simulink model "untitled"  (R2022a)
settings: Solver=VariableStepAuto  StartTime=0.0  StopTime=10  RelTol=1e-3
values from neighbouring files (symbols this model uses):
  C_PM = 1.758e-3    (= 0.001758)    [journal.m]
  Cfilter = 1/(Larm*wc2)    (= 4.78421193241e-05)    [journal.m]
  Cg = 50e-9    (= 5e-08)    [journal.m]
  Fc = Fnom*3.37    (= 168.5)    [journal.m]
  Fnom = 50    [journal.m]
  Inom = Pnom/(sqrt(3)*Vnom_dc)    [journal.m]
  Ki_Ireg = 6    [journal.m]
  Ki_Preg = 1.0    (= 1)    [journal.m]
  Ki_Qreg = 1.0    (= 1)    [journal.m]
  Ki_VDCreg = 100    [journal.m]
  Kp_Ireg = 0.6    [journal.m]
  Kp_Preg = 0.5/3    (= 0.166666666667)    [journal.m]
  Kp_Qreg = 0.5/3    (= 0.166666666667)    [journal.m]
  Kp_VDCreg = 4    [journal.m]
  L_cable = 15e-3    (= 0.015)    [journal.m]
  Larm = Larm_pu*(Zbase/(2*pi*Fnom))    (= 0.0529455974536)    [journal.m]
  Lff = Larm_pu/2    (= 0.075)    [journal.m]
  Lfilter = 0    [journal.m]
  Limits_Ireg = [ 2.0  -2.0]    [journal.m]
  Limits_Preg = [ 1.2, 0.8 ]    [journal.m]
  Limits_Qreg = [ 0.25, -0.25 ]    [journal.m]
  Limits_VDCreg = [ 2.0  -2.0]    [journal.m]
  Lxfo = 0.12    [journal.m]
  Nb_PM = 36    [journal.m]
  Pnom = 1000e6    (= 1000000000)    [journal.m]
  R_cable = 0.5    [journal.m]
  R_startup = 400    [journal.m]
  Rarm = Rarm_pu*Zbase    (= 0.1663335)    [journal.m]
  Rff = Rarm_pu/2    (= 0.00075)    [journal.m]
  Rfilter = 1/(Cfilter*w)*30    (= 1996.002)    [journal.m]
  Rg = 100    [journal.m]
  Rxfo = 0.003    [journal.m]
  Slope_Pref = 0.5    [journal.m]
  Slope_Qref = 0.5    [journal.m]
  Slope_Vdc_ref = Vnom_dc/5    (= 128000)    [journal.m]
  Tbrk1_On = 0.1    [journal.m]
  Tbrk2_On = 0.5    [journal.m]
  Tdeblock = 1    [journal.m]
  Tfault = 999    [journal.m]
  Ton_Converter2 = 2    [journal.m]
  Ton_PQreg = 2    [journal.m]
  Ton_VDCreg = 1    [journal.m]
  Ts = Ts_Control    (= 4e-05)    [journal.m]
  Ts_Control = 40e-6    (= 4e-05)    [journal.m]
  Ts_Power = 20e-6    (= 2e-05)    [journal.m]
  Vnom_dc = 640e3    (= 640000)    [journal.m]
  Vnom_prim = 400e3    (= 400000)    [journal.m]
  Vnom_sec = 333e3    (= 333000)    [journal.m]
undefined symbols (not defined in the file or in its folder): D11, Delta, DiscIntNeverNeededParam, find_system, Pcc, sigbuilder_block
libraries: powerlib_extras x42, spsSeriesRLCBranchLib x32, spsCurrentMeasurementLib x24, simulink x18, spsVoltageMeasurementLib x16, spsHalfBridgeMMCLib x12, spsThreePhaseVIMeasurementLib x10, simulink_extras x6, spsBreakerLib x6, spsParallelRLCBranchLib x6, spsThreePhaseBreakerLib x4, spsMeanLib x4
(part 1 of 6)
settings Model: SimulationMode=accelerator  Creator=Hai  LastModifiedBy=Hai

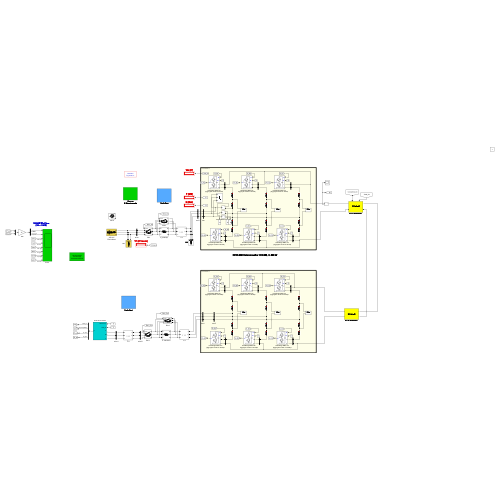
[thumbnail: Simulink's stored preview of the top-level diagram]
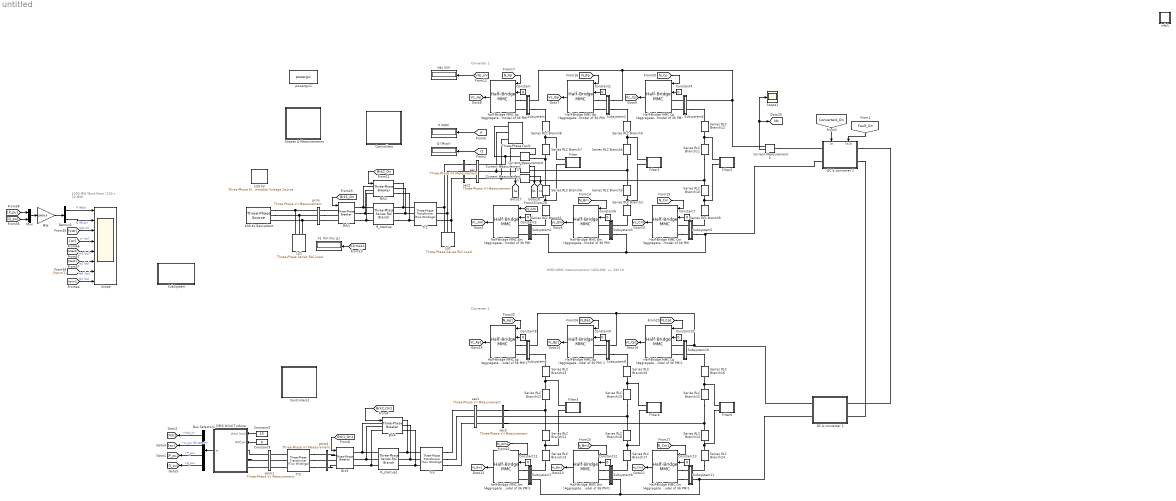
== system untitled ==
  note: HVDC-MMC Interconnection 1000-MW, +/- 320 kV
  note: Converter 1
  note: Converter 1
  note: 1000 MW Wind Farm
      | (100 x 10 MW)
  120 kV : spsThreePhaseProgrammableVoltageSourceLib/Three-Phase Programmable Voltage Source  PositiveSequence=[400e3 0 50]  VariationEntity=Amplitude  VariationType=Table of time-amplitude pairs  VariationTypeAlt=Step  VariationStep=-0.2  VariationRate=10  VariationMagnitude=0.3  VariationFrequency=2  VariationTiming=[0.05 0.05+5/60]  VariationPhaseA=off  Amplitudes=[1 0.4 1.0]  TimeValues=[0 7 7.5]  HarmonicGeneration=off  HarmonicA=[1 -0.1 0 2]  HarmonicB=[2 0.15 35 2]*0  Timing="[0.1  2]"  BusType=swing  Pref=0  Qref=0  Qmin=-inf  Qmax=inf
  400-kV Equivalent : spsThreePhaseSourceLib/Three-Phase Source  InternalConnection=Yg  VoltagePhases=off  Voltage=Vnom_prim*0.99  PhaseAngle=0  Voltage_phases=[25e3 25e3 25e3]/sqrt(3)  PhaseAngles_phases=[0 -120 +120]  Frequency=Fnom  NonIdealSource=on  SpecifyImpedance=on  Resistance=0.8929  Inductance=16.58e-3  ShortCircuitLevel=Psc  BaseVoltage=Vnom_prim  XRratio=7  BusType=swing  Pref=0  Qref=0  Prefabc=[10e3, 10e3, 10e3]  Qrefabc=[0, 0, 0]  Qmin=-inf  Qmax=inf
  Brk1 : spsThreePhaseBreakerLib/Three-Phase Breaker  InitialState=open  SwitchA=on  SwitchB=on  SwitchC=on  SwitchTimes=0.1  External=on  BreakerResistance=0.001  SnubberResistance=1e6  SnubberCapacitance=inf  Measurements=None
  Brk2 : spsThreePhaseBreakerLib/Three-Phase Breaker  InitialState=open  SwitchA=on  SwitchB=on  SwitchC=on  SwitchTimes=[30/60]*10000  External=on  BreakerResistance=0.01  SnubberResistance=1e6  SnubberCapacitance=inf  Measurements=None
  Brk3 : spsThreePhaseBreakerLib/Three-Phase Breaker  InitialState=open  SwitchA=on  SwitchB=on  SwitchC=on  SwitchTimes=0.1  External=on  BreakerResistance=0.001  SnubberResistance=1e6  SnubberCapacitance=inf  Measurements=None
  Brk4 : spsThreePhaseBreakerLib/Three-Phase Breaker  InitialState=open  SwitchA=on  SwitchB=on  SwitchC=on  SwitchTimes=[30/60]*10000  External=on  BreakerResistance=0.01  SnubberResistance=1e6  SnubberCapacitance=inf  Measurements=None
  Bus Selector1 : BusSelector  OutputSignals=Vdc_V,wr_pu (IG speed),PQ_pu.P_pu,PQ_pu.Q_pu
  Constant{,1,3..13} (13 alike) : Constant  Value=0
  Constant2 : Constant  Value=15
  Controllers : Subsystem
  Controllers1 : Subsystem
  Current Measurement{,1..3} (4 alike) : spsCurrentMeasurementLib/Current Measurement  PhasorSimulation=off  OutputType=Complex  PSBequivalent=0
  DC & converter 1 : Subsystem
      mask Display: disp('DC circuit')
  DC & converter 2 : Subsystem
      settings: PortSchema="{\"entries\":[{\"content\":{\"sides\":[{\"content\":{\"connectorIds\":[\"LConn1\",\"LConn2\"]},\"type\":\"ConnectorPlacement.EquallySpacedRectSide\",\"uuid\":\"7a2c87ad-91de-4512-ad2a-35713ffc2c67\"},{\"content\":{\"connectorIds\":[\"RConn1\",\"RConn2\"],\"side\":\"RIGHT\"},\"type\":\"ConnectorPlacement.EquallySpacedRectSide\",\"uuid\":\"a4d51b8d-9b80-4f56-8990-d227af10d4d9\"},{\"content\":{\"connectorIds\":[\"In1\",\"In2\"],\"side\":\"TOP\"},\"type\":\"ConnectorPlacement.EquallySpacedRectSide\",\"uuid\":\"21e823e1-439d-404c-83ef-6279f9df48a0\"}]},\"type\":\"ConnectorPlacement.EquallySpacedConnector\",\"uuid\":\"7be36849-7bc6-4892-aa95-a5e675f45e41\"}],\"packageUris\":[\"http://schema.mathworks.com/mf0/Connector/R2020b\"],\"version\":\"1.0\"}"
      mask Display: disp('DC circuit')
  DFIG Wind Turbine : Subsystem  LoadFcn=%find_system(gcs,'FollowLinks', 'on', 'LookUnderMasks', 'all');  mask(DFIG Wind Turbine){Nb_wt=666, ShowParameters=Generator data for 1 wind turbine, nom=[1.5e6/.9 575 1975 50], sta=[ 0.023 0.18], rot=[ 0.016 0.16], Lm=2.9, mec=[0.685 0.01 3], init=[ -0.2,0   0,0,0   0,0,0 ], Imax_grid_conv=0.8, RL_grid=[ 0.3 0.003], Vdc_nom=1150, C_DClink1=10000e-6, C_var_filter1=120e3, Pmec1=1.5e6, wind_speed_CpMax=11, wind0=11, DisplayTurbChar=off, H_WT=4.32, Ksh=1.11, D_mutual=1.5, w_wt0=1.2, torque0=0.83, Kdc=[8   400], Kgrid_side_cur_reg=[0.83 5], Kspeed=[3 0.6], Krotor_side_cur_reg=[0.6 8], Ki_QV=[0.05 20], Kp_pitch=[150], Kcompensation=[3 30], pitch_max=27, pitch_rate=10}
      mask prompts: Nb_wt "Number of wind turbines:"; ShowParameters "Display:"; nom "Nom. power, L-L volt. and freq. [Pn (VA), Vs_nom (Vrms), Vr_nom (Vrms), fn (Hz)]:"; sta "Stator [ Rs,Lls ] (p.u.):"; rot "Rotor [ Rr',Llr' ] (p.u.):"; Lm "Magnetizing inductance Lm (p.u.):"; mec "Inertia constant, friction factor, and pairs of poles [ H(s)  F(p.u.)  p ]:"; init "Initial conditions [s  th  ias  ibs  ics  phaseas phasebs phasecs]:"; Imax_grid_conv "Grid-side converter maximum current (pu of generator nominal current):"; RL_grid "Grid-side coupling inductor [ L, R] (p.u.):"; Vdc_nom "Nominal DC bus voltage (V):"; C_DClink1 "DC bus capacitor (F):"; C_var_filter1 "Line filter capacitor (Q=50) (var):"; Pmec1 "Nominal mechanical output power (W):"; wind_speed_CpMax "Wind speed at nominal speed and at Cp max (must be between 6 m/s and 30 m/s) (m/s):"; wind0 "Initial wind speed (m/s):"; DisplayTurbChar "Display wind turbine power characteristics:"; H_WT "Wind turbine inertia constant H (s):"; Ksh "Shaft spring constant refer to high-speed shaft (pu of nominal mechanical torque/rad):"; D_mutual "Shaft mutual damping (pu of nominal mechanical torque/pu dw):"; w_wt0 "Turbine initial speed (pu of nominal speed):"; torque0 "Initial output torque (pu of nominal mechanical torque):"; Kdc "DC bus voltage regulator gains [Kp Ki]:"; Kgrid_side_cur_reg "Grid-side converter current regulator gains [Kp Ki]:"; Kspeed "Speed regulator gains [Kp Ki]:"; Krotor_side_cur_reg "Rotor-side converter current regulator gains [Kp Ki]:"; Ki_QV "Q and V regulator gains [Ki_var Ki_volt]:"; Kp_pitch "Pitch controller gain [Kp]:"; Kcompensation "Pitch compensation gains [Kp Ki]:"; pitch_max "Maximum pitch angle (deg):"; pitch_rate "Maximum rate of change of pitch angle (deg/s):"
      mask help: This block implements a model of a variable speed pitch controlled wind turbine using a doubly-fed induction generator (DFIG).
      mask init:
      | %Generator data
      | Pnom=nom(1)*Nb_wt;
      | Vnom=nom(2);
      | Vnom_r=nom(3);
      | Fnom=nom(4);
      | Rs=sta(1);
      | Lls=sta(2);
      | Rr=rot(1);
      | Llr=rot(2);
      | H=mec(1);
      | F=mec(2);
      | p=mec(3);
      | 
      | % Converters data
      | L_RL=RL_grid(1);
      | R_RL=RL_grid(2);
      | Q_filter=50;
      | C_DClink=C_DClink1*Nb_wt;
      | C_var_filter=C_var_filter1*Nb_wt;
      | 
      | % Controller data
      | Freq_filter=1000*10;   %Hz
      | Zeta_filter=0.707;
      | Mod_index_max_grid=1.1;   %Maximum value of modulation index for grid-side converter
      | Mod_index_max_rotor=2;   %Maximum value of modulation index for rotor-side converter
      | Lim_grid_side_cur_reg=1.1; %Limit for grid-side PI current regulator (pu)
      | Lim_rotor_side_cur_reg=0.1; %Limit for rotor-side PI current regulator (pu)
      | Min_var_reg=0.9; %Minimum output value for integral var regulator (pu)
      | Max_var_reg=1.1; %Maximum output value for integral var regulator (pu)
      | Max_speed_reg=1; %Maximum output value for PI speed regulator (pu)
      | Kp_dc=Kdc(1);
      | Ki_dc=Kdc(2);
      | Kp_grid_side_cur_reg=Kgrid_side_cur_reg(1);
      | Ki_grid_side_cur_reg=Kgrid_side_cur_reg(2);
      | Kp_speed=Kspeed(1);
      | Ki_speed=Kspeed(2);
      | Kp_compensation=Kcompensation(1);
      | Ki_compensation=Kcompensation(2);
      | Kp_rotor_side_cur_reg=Krotor_side_cur_reg(1);
      | Ki_rotor_side_cur_reg=Krotor_side_cur_reg(2);
      | Ki_var=Ki_QV(1);
      | Ki_volt=Ki_QV(2);
      | Iq_ref_limit_time_constant=0.3; %(s)
      | T_speed=5;      %s
      | Min_mag_flux=0.5;   %(pu)
      | Max_Idr_ref=0.9;    %(pu)
      | Speed_max=1.2;  %(pu)
      | Speed_min=0.7;  %(pu)
      | Pitch_time_constant=0.01;    %(s)
      | 
      | 
      | % Turbine data
      | Pmec=Pmec1*Nb_wt;
      | c1 = 0.6450;
      | c2 = 116;
      | c3 = .4;
      | c4 = 5;
      | c5 = 21;
      | c6 = .00912;  % Set Pmin in stall condition (does not vary with wind_speed_Pmax)
      | c7 = .08;
      | c8 = .035;
      | theta=0;
      | CpMax=.5;
      | lambda_CpMax=9.9495;
      | 
      | c1_c8=[c1 c2 c3 c4 c5 c6 c7 c8];
      |   
      | 
      | %   Cp = c1*(c6*lambda + (-c4 - c3*(2.5 + theta) + c2*(1/(lambda + ...
      | %   c7*(2.5 + theta)) - c8/(1 + (2.5 + theta)^3)))/exp(c5*(1/(lambda + ...
      | %   c7*(2.5 + theta)) - c8/(1 + (2.5 + theta)^3))))
      | 
      | 
      |         %%%%%%%%%%%%%%%%%%%%%%%%%%%%%%%%%%%%%%%%%%%%%%%%%%%%%%%%%%%%%%%%%%%%%%%%%%%
      |         % Operation at Cp max
      |         %%%%%%%%%%%%%%%%%%%%%%%%%%%%%%%%%%%%%%%%%%%%%%%%%%%%%%%%%%%%%%%%%%%%%%%%%%%
      |         
      |         rated_omegar=1.2;
      |         omegar = rated_omegar;
      |         
      |         % Enforce boundaries on wind speed
      |         % A warning could be displayed
      |         if wind_speed_CpMax < 6
      |             wind_speed_CpMax=6;
      |             disp('Warning: Wind speed at nominal speed and at Cp max has been set to 6 m/s')
      |         end
      |         if wind_speed_CpMax > 30
      |             wind_speed_CpMax=30;
      |             disp('Warning: Wind speed at nominal speed and at Cp max has been set to 30 m/s')
      |         end
      | 
      |         K1=lambda_CpMax/omegar*wind_speed_CpMax;
      |         
      |         % Calculation of K2 needed to get P equal to the requested value at
      |         % Cp max for the requested wind speed
      |         
      |         Prated=Pmec1*Nb_wt;
      |         P_rated_omegar_theta_zero=0.75;
      |         
      |         K2 = P_rated_omegar_theta_zero*Prated/(wind_speed_CpMax^3*CpMax);
      |         
      |         K1_K2=[K1 K2];
      |         
      |         %%%%%%%%%%%%%%%%%%%%%%%%%%%%%%%%%%%%%%%%%%%%%%%%%%%%%%%%%%%%%%%%%%%%%%%%%%%
      |         % End of calculation for operation at Cp max
      |         %%%%%%%%%%%%%%%%%%%%%%%%%%%%%%%%%%%%%%%%%%%%%%%%%%%%%%%%%%%%%%%%%%%%%%%%%%%
      |         
      | 
      | %%%%%%%%%%%%%%%%%%%%%%%%%%%%%%%%%%%%%%%%%%%%%%%%%%%%%%%%%%%%%%%%%%%%%%%%%%%
      | % Plot turbine characteristics
      | %%%%%%%%%%%%%%%%%%%%%%%%%%%%%%%%%%%%%%%%%%%%%%%%%%%%%%%%%%%%%%%%%%%%%%%%%%% 
      | 
      | DisplayTurbChar=get_param(gcb,'DisplayTurbChar');
      | if strcmp(DisplayTurbChar,'on')
      |     vect_theta = 0:2:30;
      |     
      |     vect_lambda = 1:0.2:30;
      |     
      |     clear Cp;
      |     
      |     for i=1:length(vect_theta)
      |      for j=1:length(vect_lambda)
      |                 Cp(i,j) = c1*(c6*vect_lambda(j) + (-c4 - c3*(2.5 + vect_theta(i)) + c2*(1/(vect_lambda(j) + ...
      |                 c7*(2.5 + vect_theta(i))) - c8/(1 + (2.5 + vect_theta(i))^3)))/exp(c5*(1/(vect_lambda(j) + ...
      |                 c7*(2.5 + vect_theta(i))) - c8/(1 + (2.5 + vect_theta(i))^3))));
      |      end
      |     end
      | 
      |     figure(1);
      |     clf;
      |     hold on;
      | 
      |     plot(vect_lambda, Cp);
      |     axis([0, 25, 0, .6]);
      |     title('Wind Turbine Cp Characteristic (pitch angle increases by step of 2 deg.)');
      |     ylabel('Cp');
      |     set(gca,'ytick',[0 .1 .2 .3 .4 .5 .6]);
      |     xlabel('Lambda');
      |     grid on;
      |     text(10.1,0.51,'Pitch angle 0 degree');
      | 
      |     hold off
      |     
      |     % Plot of the wind turbine mechanical power output (pu) lambda and Cp
      |     % characteristics against wind speed (m/s) for a range of theta.
      |     
      |     wind_speed_range = [1,.2,30];
      |     vect_wind_speed = 1:0.2:30;
      |     
      |     clear lambda;
      |     clear Cp;
      |     clear P;
      | 
      |     for i=1:length(vect_theta)
      |         for j=1:length(vect_wind_speed)
      |             lambda(i,j) = K1*omegar/vect_wind_speed(j);
      |             Cp(i,j) = c1*(c6*lambda(i,j) + (-c4 - c3*(2.5 + vect_theta(i)) + c2*(1/(lambda(i,j) + ...
      |             c7*(2.5 + vect_theta(i))) - c8/(1 + (2.5 + vect_theta(i))^3)))/exp(c5*(1/(lambda(i,j) + ...
      |             c7*(2.5 + vect_theta(i))) - c8/(1 + (2.5 + vect_theta(i))^3))));
      |             P(i,j) = K2/Prated*vect_wind_speed(j)^3*Cp(i,j);
      |         end
      |     end
      |     
      |     
      |     figure(2);
      |     clf;
      |     hold on
      |     
      |     subplot(3,1,1);
      |     plot(vect_wind_speed, P);
      |     axis([0, 35, 0, 1.5]);
      |     title('Wind Turbine Characteristics (w = 1.2 pu, pitch angle increases by step of 2 deg.)');
      |     ylabel('P (pu)');
      |     set(gca,'ytick',0:.5:4);
      |     grid on;
      |     
      |     subplot(3,1,2);
      |     plot(vect_wind_speed, lambda);
      |     axis([0, 35, 0, 20]);
      |     ylabel('Lambda');
      |     grid on;
      |     
      |     subplot(3,1,3)
      |     plot(vect_wind_speed, Cp);
      |     axis([0, 35, 0, .6]);
      |     xlabel('Wind Speed (m/s)');
      |     ylabel('Cp');
      |     set(gca,'ytick',[0 .1 .2 .3 .4 .5 .6]);
      |     grid on;
      | 
      |     hold off
      |     set_param(gcb,'DisplayTurbChar','off')
      |     
      | end
      mask TypeOptions ShowParameters: Generator data for 1 wind turbine | Converters data for 1 wind turbine | Turbine data for 1 wind turbine | Drive train data for 1 wind turbine | Control parameters for 1 wind turbine
      mask Callback ShowParameters:
      | BlockName=getfullname(gcb);
      | %
      | Param_Show=get_param(BlockName,'ShowParameters');
      | Param_DisplayTurbChar=get_param(BlockName,'DisplayTurbChar');
      | 
      | p_mask{3}='off';p_mask{4}='off';p_mask{5}='off';
      | p_mask{6}='off';p_mask{7}='off';p_mask{8}='off';p_mask{9}='off';
      | p_mask{10}='off';p_mask{11}='off';p_mask{12}='off';p_mask{13}='off';
      | p_mask{14}='off';p_mask{15}='off';p_mask{16}='off';p_mask{17}='off';
      | p_mask{18}='off';p_mask{19}='off';p_mask{20}='off';p_mask{21}='off';
      | p_mask{22}='off';p_mask{23}='off';p_mask{24}='off';p_mask{25}='off';
      | p_mask{26}='off';p_mask{27}='off';p_mask{28}='off';p_mask{29}='off';
      | p_mask{30}='off';p_mask{31}='off';
      | 
      | 
      | switch Param_Show
      | 	case 'Generator data for 1 wind turbine'
      | 		p_mask{3}='on';p_mask{4}='on';p_mask{5}='on'; p_mask{6}='on';
      |         p_mask{7}='on'; p_mask{8}='on';
      |     case 'Converters data for 1 wind turbine'
      | 		p_mask{9}='on';p_mask{10}='on';p_mask{11}='on';p_mask{12}='on';
      |         p_mask{13}='on';
      | 	case 'Turbine data for 1 wind turbine'
      |         p_mask{14}='on';p_mask{15}='on';p_mask{16}='on';p_mask{17}='on';
      |     case 'Drive train data for 1 wind turbine'
      |         p_mask{18}='on';p_mask{19}='on';p_mask{20}='on';p_mask{21}='on';
      |         p_mask{22}='on';
      |     case 'Control parameters for 1 wind turbine'
      |         p_mask{23}='on';p_mask{24}='on';p_mask{25}='on';
      |         p_mask{26}='on';p_mask{27}='on';p_mask{28}='on';p_mask{29}='on';
      |         p_mask{30}='on'; p_mask{31}='on';
      | end
      | 
      | ParVisible={'on','on',p_mask{3},p_mask{4},p_mask{5},p_mask{6},p_mask{7},...
      |     p_mask{8},p_mask{9},p_mask{10},p_mask{11},p_mask{12},p_mask{13},...
      |     p_mask{14},p_mask{15},p_mask{16},p_mask{17},p_mask{18},p_mask{19},...
      |     p_mask{20},p_mask{21},p_mask{22},p_mask{23},p_mask{24},p_mask{25},...
      |     p_mask{26},p_mask{27},p_mask{28},p_mask{29},p_mask{30},p_mask{31},...
      |     };
      | %
      | set_param(BlockName,'MaskVisibilities',ParVisible);
      | set_param(BlockName,'DisplayTurbChar',Param_DisplayTurbChar);
  Demux2 : Demux  Outputs=2
  Filter : Subsystem
      mask Display: disp('Filter')
  Filter1 : Subsystem
      mask Display: disp('Filter')
  Filter2 : Subsystem
      mask Display: disp('Filter')
  Filter3 : Subsystem
      mask Display: disp('Filter')
  Filter4 : Subsystem
      mask Display: disp('Filter')
  Filter5 : Subsystem
      mask Display: disp('Filter')
  Half-Bridge MMC Am (Aggregate model of 36 PM) : spsHalfBridgeMMCLib/Half-Bridge MMC  ModelType=Aggregate model  n=36  C=C_PM  Vc_Initial=Vc0_PM  Ron=1e-3  Rs=1e6  Cs=inf  Ron_Diode=1e-3  Rs_Diode=1e6  Cs_Diode=inf  Vf_Diode=1e-3  Rs_CurrentSource=inf  Ts=Ts_Power
      settings: SourceProductBaseCode=PS
  Half-Bridge MMC Am (Aggregate model of 36 PM)1 : spsHalfBridgeMMCLib/Half-Bridge MMC  ModelType=Aggregate model  n=36  C=C_PM  Vc_Initial=Vc0_PM  Ron=1e-3  Rs=1e6  Cs=inf  Ron_Diode=1e-3  Rs_Diode=1e6  Cs_Diode=inf  Vf_Diode=1e-3  Rs_CurrentSource=inf  Ts=Ts_Power
      settings: SourceProductBaseCode=PS
  Half-Bridge MMC Ap (Aggregate model of 36 PM) : spsHalfBridgeMMCLib/Half-Bridge MMC  ModelType=Aggregate model  n=36  C=C_PM  Vc_Initial=Vc0_PM  Ron=1e-3  Rs=1e6  Cs=inf  Ron_Diode=1e-3  Rs_Diode=1e6  Cs_Diode=inf  Vf_Diode=1e-3  Rs_CurrentSource=inf  Ts=Ts_Power
      settings: SourceProductBaseCode=PS
  Half-Bridge MMC Ap (Aggregate model of 36 PM)1 : spsHalfBridgeMMCLib/Half-Bridge MMC  ModelType=Aggregate model  n=36  C=C_PM  Vc_Initial=Vc0_PM  Ron=1e-3  Rs=1e6  Cs=inf  Ron_Diode=1e-3  Rs_Diode=1e6  Cs_Diode=inf  Vf_Diode=1e-3  Rs_CurrentSource=inf  Ts=Ts_Power
      settings: SourceProductBaseCode=PS
  Half-Bridge MMC Bm (Aggregate model of 36 PM) : spsHalfBridgeMMCLib/Half-Bridge MMC  ModelType=Aggregate model  n=36  C=C_PM  Vc_Initial=Vc0_PM  Ron=1e-3  Rs=1e6  Cs=inf  Ron_Diode=1e-3  Rs_Diode=1e6  Cs_Diode=inf  Vf_Diode=1e-3  Rs_CurrentSource=inf  Ts=Ts_Power
      settings: SourceProductBaseCode=PS
  Half-Bridge MMC Bm (Aggregate model of 36 PM)1 : spsHalfBridgeMMCLib/Half-Bridge MMC  ModelType=Aggregate model  n=36  C=C_PM  Vc_Initial=Vc0_PM  Ron=1e-3  Rs=1e6  Cs=inf  Ron_Diode=1e-3  Rs_Diode=1e6  Cs_Diode=inf  Vf_Diode=1e-3  Rs_CurrentSource=inf  Ts=Ts_Power
      settings: SourceProductBaseCode=PS
  "Half-Bridge MMC Bp (Aggregate model of 36 PM) " : spsHalfBridgeMMCLib/Half-Bridge MMC  ModelType=Aggregate model  n=36  C=C_PM  Vc_Initial=Vc0_PM  Ron=1e-3  Rs=1e6  Cs=inf  Ron_Diode=1e-3  Rs_Diode=1e6  Cs_Diode=inf  Vf_Diode=1e-3  Rs_CurrentSource=inf  Ts=Ts_Power
      settings: SourceProductBaseCode=PS
  Half-Bridge MMC Bp (Aggregate model of 36 PM) 1 : spsHalfBridgeMMCLib/Half-Bridge MMC  ModelType=Aggregate model  n=36  C=C_PM  Vc_Initial=Vc0_PM  Ron=1e-3  Rs=1e6  Cs=inf  Ron_Diode=1e-3  Rs_Diode=1e6  Cs_Diode=inf  Vf_Diode=1e-3  Rs_CurrentSource=inf  Ts=Ts_Power
      settings: SourceProductBaseCode=PS
  Half-Bridge MMC Cm (Aggregate model of 36 PM) : spsHalfBridgeMMCLib/Half-Bridge MMC  ModelType=Aggregate model  n=36  C=C_PM  Vc_Initial=Vc0_PM  Ron=1e-3  Rs=1e6  Cs=inf  Ron_Diode=1e-3  Rs_Diode=1e6  Cs_Diode=inf  Vf_Diode=1e-3  Rs_CurrentSource=inf  Ts=Ts_Power
      settings: SourceProductBaseCode=PS
  Half-Bridge MMC Cm (Aggregate model of 36 PM)1 : spsHalfBridgeMMCLib/Half-Bridge MMC  ModelType=Aggregate model  n=36  C=C_PM  Vc_Initial=Vc0_PM  Ron=1e-3  Rs=1e6  Cs=inf  Ron_Diode=1e-3  Rs_Diode=1e6  Cs_Diode=inf  Vf_Diode=1e-3  Rs_CurrentSource=inf  Ts=Ts_Power
      settings: SourceProductBaseCode=PS
  Half-Bridge MMC Cp (Aggregate model of 36 PM) : spsHalfBridgeMMCLib/Half-Bridge MMC  ModelType=Aggregate model  n=36  C=C_PM  Vc_Initial=Vc0_PM  Ron=1e-3  Rs=1e6  Cs=inf  Ron_Diode=1e-3  Rs_Diode=1e6  Cs_Diode=inf  Vf_Diode=1e-3  Rs_CurrentSource=inf  Ts=Ts_Power
      settings: SourceProductBaseCode=PS
  Half-Bridge MMC Cp (Aggregate model of 36 PM)1 : spsHalfBridgeMMCLib/Half-Bridge MMC  ModelType=Aggregate model  n=36  C=C_PM  Vc_Initial=Vc0_PM  Ron=1e-3  Rs=1e6  Cs=inf  Ron_Diode=1e-3  Rs_Diode=1e6  Cs_Diode=inf  Vf_Diode=1e-3  Rs_CurrentSource=inf  Ts=Ts_Power
      settings: SourceProductBaseCode=PS
  Ld1 : spsThreePhaseSeriesRLCLoadLib/Three-Phase Series RLC Load  LConnTagsString=A|B|C  Configuration=Y (grounded)  NominalVoltage=Vnom_prim  Vabc=[1e3 1e3 1e3]  Vabcp=[1e3 1e3 1e3]  NominalFrequency=Fnom  UnbalancedPower=off  ActivePower=P_Ld1  InductivePower=0  CapacitivePower=0  Pabc=[10e3 9e3 11e3]  QLabc=[100 90 110]  QCabc=[100 90 110]  Pabcp=[10e3 9e3 11e3]  QLabcp=[100 90 110]  QCabcp=[100 90 110]  Measurements=None  LoadType=constant Z
  Ld2 : spsThreePhaseSeriesRLCLoadLib/Three-Phase Series RLC Load  LConnTagsString=A|B|C  Configuration=Y (grounded)  NominalVoltage=Vnom_sec  Vabc=[1e3 1e3 1e3]  Vabcp=[1e3 1e3 1e3]  NominalFrequency=Fnom  UnbalancedPower=off  ActivePower=500e3  InductivePower=0  CapacitivePower=0  Pabc=[10e3 9e3 11e3]  QLabc=[100 90 110]  QCabc=[100 90 110]  Pabcp=[10e3 9e3 11e3]  QLabcp=[100 90 110]  QCabcp=[100 90 110]  Measurements=None  LoadType=constant Z
  MW : Gain  Gain=1000/0.9  SaturateOnIntegerOverflow=on  OutDataTypeStr=Inherit: Same as input  ParamDataTypeStr=Inherit: Same as input
  Mux : Mux  Inputs=2
  P (MW) : Display
      settings: Format=bank  Decimation=5000
  Q (Mvar) : Display
      settings: Format=bank  Decimation=5000
  R_startup : spsThreePhaseSeriesRLCBranchLib/Three-Phase Series RLC Branch  LConnTagsString=A|B|C  RConnTagsString=A|B|C  BranchType=R  Resistance=R_startup  Inductance=Vnom_prim^2 / Pcc / (2*pi*Fnom)  Capacitance=1e-6  Measurements=None
  R_startup1 : spsThreePhaseSeriesRLCBranchLib/Three-Phase Series RLC Branch  LConnTagsString=A|B|C  RConnTagsString=A|B|C  BranchType=R  Resistance=R_startup  Inductance=Vnom_prim^2 / Pcc / (2*pi*Fnom)  Capacitance=1e-6  Measurements=None
  Scope : Scope  NumInputPorts=8
  Scope1 : Scope
  Scopes & Measurements : Subsystem
  Series RLC Branch{1..24} (24 alike) : spsSeriesRLCBranchLib/Series RLC Branch  LConnTagsString=__new0  RConnTagsString=__new0  BranchType=RL  Resistance=Rarm/2  Inductance=Larm/2  SetiL0=off  InitialCurrent=0  Capacitance=1e-6  Setx0=off  InitialVoltage=0  Measurements=None
  SubSystem : Subsystem
      settings: OpenFcn=openfig('power_wind_dfig_DetVsAvg.fig');
      mask Display: disp('Show Detailed\n and Average\n Simulation Results')
  Subsystem : Subsystem
  Subsystem1 : Subsystem
  Subsystem10 : Subsystem
  Subsystem11 : Subsystem
  Subsystem2 : Subsystem
  Subsystem3 : Subsystem
  Subsystem4 : Subsystem
  Subsystem5 : Subsystem
  Subsystem6 : Subsystem
  Subsystem7 : Subsystem
  Subsystem8 : Subsystem
  Subsystem9 : Subsystem
  Three-Phase Fault : spsThreePhaseFaultLib/Three-Phase Fault  InitialStates=0  FaultA=on  FaultB=off  FaultC=off  GroundFault=on  SwitchTimes="[7  7+0.5]"  External=off  SwitchStatus=NaN  FaultResistance=0.0005*2  GroundResistance=0.005*2  SnubberResistance=1e6  SnubberCapacitance=inf  Measurements=None
  Tr1 : spsThreePhaseTransformerTwoWindingsLib/Three-Phase Transformer (Two Windings)  Winding1Connection=Yg  Winding2Connection=Delta (D11)  CoreType=Three single-phase transformers  SetSaturation=off  Hysteresis=off  DataFile='hysteresis'  SetInitialFlux=off  Measurements=None  UNITS=pu  NominalPower=[ Pnom , Fnom ]  Winding1="[ Vnom_prim , Rxfo/2,  Lxfo/2 ]"  Winding2="[ Vnom_sec , Rxfo/2,  Lxfo/2 ]"  Rm=1000  Lm=1000  L0=0.5  Saturation=[ 0,0 ; 0.0024,1.2 ; 1.0,1.52 ]  InitialFluxes=[ 0.8 , -0.8 , 0.7 ]  BreakLoop=off  DiscreteSolver=Trapezoidal iterative  DataType=off  TransfoNumber=1
  Tr2 : spsThreePhaseTransformerTwoWindingsLib/Three-Phase Transformer (Two Windings)  Winding1Connection=Yg  Winding2Connection=Yg  CoreType=Three single-phase transformers  SetSaturation=off  Hysteresis=off  DataFile='hysteresis'  SetInitialFlux=off  Measurements=None  UNITS=pu  NominalPower=[ Pnom , Fnom ]  Winding1="[2345, Rxfo/2,  Lxfo/2 ]"  Winding2="[ Vnom_prim , Rxfo/2,  Lxfo/2 ]"  Rm=1000  Lm=1000  L0=0.5  Saturation=[ 0,0 ; 0.0024,1.2 ; 1.0,1.52 ]  InitialFluxes=[ 0.8 , -0.8 , 0.7 ]  BreakLoop=off  DiscreteSolver=Trapezoidal iterative  DataType=off  TransfoNumber=1
  Tr3 : spsThreePhaseTransformerTwoWindingsLib/Three-Phase Transformer (Two Windings)  Winding1Connection=Yg  Winding2Connection=Delta (D11)  CoreType=Three single-phase transformers  SetSaturation=off  Hysteresis=off  DataFile='hysteresis'  SetInitialFlux=off  Measurements=None  UNITS=pu  NominalPower=[ Pnom , Fnom ]  Winding1="[Vnom_prim , Rxfo/2,  Lxfo/2 ]"  Winding2="[ Vnom_sec , Rxfo/2,  Lxfo/2 ]"  Rm=1000  Lm=1000  L0=0.5  Saturation=[ 0,0 ; 0.0024,1.2 ; 1.0,1.52 ]  InitialFluxes=[ 0.8 , -0.8 , 0.7 ]  BreakLoop=off  DiscreteSolver=Trapezoidal iterative  DataType=off  TransfoNumber=1
  V1 (kV rms LL) : Display
      settings: Format=bank  Decimation=5000
  Vdc (kV) : Display
      settings: Format=bank  Decimation=5000
  info1 : Subsystem
      settings: OpenFcn=showdemo(bdroot(gcb))
      mask Display: disp('?')
  powergui1 : spspowerguiLib/powergui  Priority=1  SimulationMode=Discrete  SampleTime=Ts_Power  frequency=60  Iterations=50  frequencyindice=0  Pbase=100e6  ErrMax=1e-4  UnitsV=kV  UnitsW=MW  buscounter=0  FunctionMessages=off  echomessages=off  EnableUseOfTLC=off  CurrentSourceSwitches=off  DisableSnubberDevices=off  DisableRonSwitches=off  DisableVfSwitches=off  DisplayEquations=off  AutomaticDiscreteSolvers=off  SolverType=Tustin/Backward Euler (TBE)  Interpol=off  ExternalGateDelay=off  methode=off  Ts=10  x0status=blocks  SPID=off  SwTol=0  HookPort=off  NonlinearTolerance=1e-4  nMaxIteration=100  ContinueOnMaxIteration=off  RestoreLinks=warning  ResistiveCurrentMeasurement=off  Frange=[0:2:500]  Ylog=off  Xlog=on  ShowGrid=off  save=off  variable=ZData  structure=VIprim  ZoomFFT=on  StartTime=0.15  cycles=2  DisplayStyle=1  fundamental=50  FreqAxis=on  MaxFrequency=1000  frequencyindicesteady=1  RmsSteady=1  display=off
  prim : spsThreePhaseVIMeasurementLib/Three-Phase V-I Measurement  VoltageMeasurement=phase-to-ground  SetLabelV=on  LabelV=Vprim  Vpu=off  VpuLL=off  CurrentMeasurement=yes  SetLabelI=on  LabelI=Iprim  Ipu=off  Pbase=100e6  Vbase=500e3  OutputType=Complex  PhasorSimulation=off  PSBequivalent=0
  prim1 : spsThreePhaseVIMeasurementLib/Three-Phase V-I Measurement  VoltageMeasurement=phase-to-ground  SetLabelV=on  LabelV=Vprim1  Vpu=off  VpuLL=off  CurrentMeasurement=yes  SetLabelI=on  LabelI=Iprim1  Ipu=off  Pbase=100e6  Vbase=500e3  OutputType=Complex  PhasorSimulation=off  PSBequivalent=0
  prim2 : spsThreePhaseVIMeasurementLib/Three-Phase V-I Measurement  VoltageMeasurement=phase-to-ground  SetLabelV=on  LabelV=Vprim2  Vpu=off  VpuLL=off  CurrentMeasurement=yes  SetLabelI=on  LabelI=Iprim2  Ipu=off  Pbase=100e6  Vbase=500e3  OutputType=Complex  PhasorSimulation=off  PSBequivalent=0
  sec : spsThreePhaseVIMeasurementLib/Three-Phase V-I Measurement  VoltageMeasurement=phase-to-ground  SetLabelV=on  LabelV=Vsec  Vpu=off  VpuLL=off  CurrentMeasurement=yes  SetLabelI=on  LabelI=Isec  Ipu=off  Pbase=100e6  Vbase=500e3  OutputType=Complex  PhasorSimulation=off  PSBequivalent=0
  sec1 : spsThreePhaseVIMeasurementLib/Three-Phase V-I Measurement  VoltageMeasurement=phase-to-ground  SetLabelV=on  LabelV=Vsec1  Vpu=off  VpuLL=off  CurrentMeasurement=yes  SetLabelI=on  LabelI=Isec1  Ipu=off  Pbase=100e6  Vbase=500e3  OutputType=Complex  PhasorSimulation=off  PSBequivalent=0
  sec2 : spsThreePhaseVIMeasurementLib/Three-Phase V-I Measurement  VoltageMeasurement=phase-to-phase  SetLabelV=on  LabelV=Vsec2  Vpu=off  VpuLL=off  CurrentMeasurement=yes  SetLabelI=on  LabelI=Isec2  Ipu=off  Pbase=100e6  Vbase=500e3  OutputType=Complex  PhasorSimulation=off  PSBequivalent=0
  sec3 : spsThreePhaseVIMeasurementLib/Three-Phase V-I Measurement  VoltageMeasurement=phase-to-phase  SetLabelV=on  LabelV=Vsec3  Vpu=off  VpuLL=off  CurrentMeasurement=yes  SetLabelI=on  LabelI=Isec3  Ipu=off  Pbase=100e6  Vbase=500e3  OutputType=Complex  PhasorSimulation=off  PSBequivalent=0
  tag scope: Ia=global, Ib=global, Ic=global, Idc=global, Vc_Am1=global, Vc_Am=global, Vc_Ap1=global, Vc_Ap=global, Vc_Bm1=global, Vc_Bm=global, Vc_Bp1=global, Vc_Bp=global, Vc_Cm1=global, Vc_Cm=global, Vc_Cp1=global, Vc_Cp=global
  wires:
  [N_Am] -> Half-Bridge MMC Am (Aggregate model of 36 PM)/1
  [Q] -> Q (Mvar)/1
  [N_Cm] -> Half-Bridge MMC Cm (Aggregate model of 36 PM)/1
  Constant/1 -> Half-Bridge MMC Ap (Aggregate model of 36 PM)/2
  "Half-Bridge MMC Bp (Aggregate model of 36 PM) "/1 -> [Vc_Bp]
  Half-Bridge MMC Cm (Aggregate model of 36 PM)/1 -> [Vc_Cm]
  Half-Bridge MMC Bm (Aggregate model of 36 PM)/1 -> [Vc_Bm]
  [N_Ap] -> Half-Bridge MMC Ap (Aggregate model of 36 PM)/1
  [Brk1_On] -> Brk1/1
  Half-Bridge MMC Ap (Aggregate model of 36 PM)/1 -> [Vc_Ap]
  [N_Bm] -> Half-Bridge MMC Bm (Aggregate model of 36 PM)/1
  [Brk2_On] -> Brk2/1
  [P] -> P (MW)/1
  [N_Cp] -> Half-Bridge MMC Cp (Aggregate model of 36 PM)/1
  Half-Bridge MMC Cp (Aggregate model of 36 PM)/1 -> [Vc_Cp]
  Half-Bridge MMC Am (Aggregate model of 36 PM)/1 -> [Vc_Am]
  [N_Bp] -> "Half-Bridge MMC Bp (Aggregate model of 36 PM) "/1
  Constant6/1 -> Half-Bridge MMC Bm (Aggregate model of 36 PM)/2
  Constant4/1 -> Half-Bridge MMC Cp (Aggregate model of 36 PM)/2
  [V1rmsLL] -> V1 (kV rms LL)/1
  Constant5/1 -> Half-Bridge MMC Am (Aggregate model of 36 PM)/2
  Constant7/1 -> Half-Bridge MMC Cm (Aggregate model of 36 PM)/2
  [Vdc_kV] -> Vdc (kV)/1
  Constant1/1 -> "Half-Bridge MMC Bp (Aggregate model of 36 PM) "/2
  Bus Selector1/4 -> [Q_pu]  "<Q_pu>"
  DFIG Wind Turbine/1(m) -> Bus Selector1/1
  Bus Selector1/1 -> [Vdc]  "<Vdc_V>"
  Bus Selector1/2 -> [wr]  "<wr_pu (IG speed)>"
  Bus Selector1/3 -> [P_pu]  "<P_pu>"
  Constant3/1 -> DFIG Wind Turbine/2(Qref_pu)
  Constant2/1 -> DFIG Wind Turbine/1("Wind (m/s) ")
  [Brk1_On1] -> Brk3/1
  [Brk2_On1] -> Brk4/1
  [N_Cp1] -> Half-Bridge MMC Cp (Aggregate model of 36 PM)1/1
  Constant11/1 -> Half-Bridge MMC Am (Aggregate model of 36 PM)1/2
  [N_Bp1] -> Half-Bridge MMC Bp (Aggregate model of 36 PM) 1/1
  [N_Bm1] -> Half-Bridge MMC Bm (Aggregate model of 36 PM)1/1
  [N_Cm1] -> Half-Bridge MMC Cm (Aggregate model of 36 PM)1/1
  Half-Bridge MMC Ap (Aggregate model of 36 PM)1/1 -> [Vc_Ap1]
  Constant9/1 -> Half-Bridge MMC Bp (Aggregate model of 36 PM) 1/2
  Half-Bridge MMC Cp (Aggregate model of 36 PM)1/1 -> [Vc_Cp1]
  Half-Bridge MMC Bp (Aggregate model of 36 PM) 1/1 -> [Vc_Bp1]
  Half-Bridge MMC Cm (Aggregate model of 36 PM)1/1 -> [Vc_Cm1]
  Constant13/1 -> Half-Bridge MMC Cm (Aggregate model of 36 PM)1/2
  [N_Ap1] -> Half-Bridge MMC Ap (Aggregate model of 36 PM)1/1
  Constant12/1 -> Half-Bridge MMC Bm (Aggregate model of 36 PM)1/2
  Half-Bridge MMC Bm (Aggregate model of 36 PM)1/1 -> [Vc_Bm1]
  Constant10/1 -> Half-Bridge MMC Cp (Aggregate model of 36 PM)1/2
  [N_Am1] -> Half-Bridge MMC Am (Aggregate model of 36 PM)1/1
  Half-Bridge MMC Am (Aggregate model of 36 PM)1/1 -> [Vc_Am1]
  Constant8/1 -> Half-Bridge MMC Ap (Aggregate model of 36 PM)1/2
  [Converter2_On] -> DC & converter 2/1(On)
  Demux2/1 -> Scope/1  "P (MW)"
  [P_pu] -> Mux/1
  Demux2/2 -> Scope/2  "Q (Mvar)"
  MW/1 -> Demux2/1
  [Vdc] -> Scope/3  "Vdc (V)"
  [Isec1] -> Scope/6  "Is1 (pu)"
  [Iprim1] -> Scope/8  "Ip1 (pu)"
  [wr] -> Scope/4  "wr (pu)"
  [Vprim1] -> Scope/7  "Vp1 (pu)"
  Mux/1 -> MW/1
  [Q_pu] -> Mux/2
  [Vsec1] -> Scope/5  "Vs1 (pu)"
  [Fault_On] -> DC & converter 2/2(Fault)
  Current Measurement/1 -> [Ia]
  Current Measurement1/1 -> [Ic]
  Current Measurement2/1 -> [Ib]
  Current Measurement3/1 -> Scope1/1, [Idc]
  connections:
  Series RLC Branch7/RConn1 -- Series RLC Branch6/LConn1 -- Current Measurement/RConn1
  Ld1/LConn1 -- 400-kV Equivalent/RConn1 -- prim/RConn1
  Ld1/LConn3 -- 400-kV Equivalent/RConn3 -- prim/RConn3
  R_startup/LConn2 -- Brk1/RConn2 -- Brk2/LConn2
  Ld1/LConn2 -- 400-kV Equivalent/RConn2 -- prim/RConn2
  Ld2/LConn3 -- sec2/RConn3 -- Tr1/RConn3
  R_startup/LConn3 -- Brk1/RConn3 -- Brk2/LConn3
  Tr1/LConn3 -- R_startup/RConn3 -- Brk2/RConn3
  Ld2/LConn1 -- sec2/RConn1 -- Tr1/RConn1
  Series RLC Branch3/RConn1 -- Filter1/LConn2 -- Series RLC Branch2/LConn1
  Ld2/LConn2 -- sec2/RConn2 -- Tr1/RConn2
  Series RLC Branch8/RConn1 -- Series RLC Branch7/LConn1 -- Filter/LConn1
  Filter2/LConn1 -- Series RLC Branch11/LConn1 -- Series RLC Branch12/RConn1
  Series RLC Branch9/LConn1 -- Filter2/LConn2 -- Series RLC Branch10/RConn1
  Three-Phase Fault/LConn3 -- Current Measurement1/LConn1 -- sec/LConn3
  Three-Phase Fault/LConn2 -- Current Measurement2/LConn1 -- sec/LConn2
  Tr1/LConn1 -- Brk2/RConn1 -- R_startup/RConn1
  Series RLC Branch6/RConn1 -- Series RLC Branch1/LConn1 -- Filter/LConn2
  Brk1/RConn1 -- Brk2/LConn1 -- R_startup/LConn1
  Series RLC Branch5/RConn1 -- Series RLC Branch4/LConn1 -- Filter1/LConn1
  Tr1/LConn2 -- R_startup/RConn2 -- Brk2/RConn2
  Series RLC Branch9/RConn1 -- Subsystem5/RConn1
  Half-Bridge MMC Cm (Aggregate model of 36 PM)/LConn1 -- Subsystem5/LConn1
  "Half-Bridge MMC Bp (Aggregate model of 36 PM) "/LConn1 -- Subsystem2/LConn1
  Subsystem/LConn2 -- Half-Bridge MMC Ap (Aggregate model of 36 PM)/LConn2
  Half-Bridge MMC Am (Aggregate model of 36 PM)/LConn1 -- Subsystem1/LConn1
  Series RLC Branch1/RConn1 -- Subsystem1/RConn1
  "Half-Bridge MMC Bp (Aggregate model of 36 PM) "/LConn2 -- Subsystem2/LConn2
  Half-Bridge MMC Bm (Aggregate model of 36 PM)/LConn1 -- Subsystem3/LConn1
  Series RLC Branch2/RConn1 -- Subsystem3/RConn1
  Subsystem/RConn2 -- Series RLC Branch8/LConn1
  Half-Bridge MMC Bm (Aggregate model of 36 PM)/LConn2 -- Subsystem3/LConn2
  Subsystem2/RConn2 -- Series RLC Branch5/LConn1
  Subsystem4/RConn2 -- Series RLC Branch12/LConn1
  Half-Bridge MMC Ap (Aggregate model of 36 PM)/LConn1 -- Subsystem/LConn1
  Half-Bridge MMC Cm (Aggregate model of 36 PM)/LConn2 -- Subsystem5/LConn2
  Half-Bridge MMC Cp (Aggregate model of 36 PM)/LConn2 -- Subsystem4/LConn2
  Half-Bridge MMC Cp (Aggregate model of 36 PM)/LConn1 -- Subsystem4/LConn1
  Half-Bridge MMC Am (Aggregate model of 36 PM)/LConn2 -- Subsystem1/LConn2
  sec2/LConn1 -- sec/RConn1
  sec2/LConn2 -- sec/RConn2
  sec2/LConn3 -- sec/RConn3
  prim/LConn1 -- Brk1/LConn1
  prim/LConn2 -- Brk1/LConn2
  prim/LConn3 -- Brk1/LConn3
  R_startup1/LConn1 -- Brk4/LConn1 -- Brk3/RConn1
  R_startup1/LConn2 -- Brk4/LConn2 -- Brk3/RConn2
  R_startup1/LConn3 -- Brk4/LConn3 -- Brk3/RConn3
  Brk4/RConn1 -- Tr3/LConn1 -- R_startup1/RConn1
  Brk4/RConn2 -- Tr3/LConn2 -- R_startup1/RConn2
  R_startup1/RConn3 -- Tr3/LConn3 -- Brk4/RConn3
  sec3/RConn2 -- sec1/LConn2
  sec3/RConn1 -- sec1/LConn1
  sec3/RConn3 -- sec1/LConn3
  Tr3/RConn1 -- sec1/RConn1
  Tr3/RConn2 -- sec1/RConn2
  Tr3/RConn3 -- sec1/RConn3
  Subsystem7/RConn2 -- Subsystem11/RConn2 -- DC & converter 1/LConn2 -- Subsystem9/RConn2
  Series RLC Branch21/RConn1 -- Filter3/LConn2 -- Series RLC Branch13/LConn1
  Series RLC Branch16/RConn1 -- Series RLC Branch15/LConn1 -- Filter5/LConn1
  Series RLC Branch23/RConn1 -- Filter3/LConn1 -- Series RLC Branch22/LConn1
  Series RLC Branch18/RConn1 -- Series RLC Branch17/LConn1 -- Filter4/LConn2
  Series RLC Branch14/RConn1 -- Filter5/LConn2 -- Series RLC Branch24/LConn1
  Subsystem6/RConn1 -- DC & converter 1/LConn1 -- Subsystem10/RConn1 -- Subsystem8/RConn1
  Filter4/LConn1 -- Series RLC Branch19/LConn1 -- Series RLC Branch20/RConn1
  Subsystem6/LConn2 -- Half-Bridge MMC Ap (Aggregate model of 36 PM)1/LConn2
  Half-Bridge MMC Bm (Aggregate model of 36 PM)1/LConn1 -- Subsystem9/LConn1
  Half-Bridge MMC Ap (Aggregate model of 36 PM)1/LConn1 -- Subsystem6/LConn1
  Half-Bridge MMC Cm (Aggregate model of 36 PM)1/LConn1 -- Subsystem11/LConn1
  Half-Bridge MMC Bp (Aggregate model of 36 PM) 1/LConn2 -- Subsystem8/LConn2
  Series RLC Branch22/RConn1 -- sec3/LConn1 -- Series RLC Branch21/LConn1
  Series RLC Branch15/RConn1 -- sec3/LConn3 -- Series RLC Branch14/LConn1
  Series RLC Branch19/RConn1 -- Series RLC Branch18/LConn1 -- sec3/LConn2
  Series RLC Branch13/RConn1 -- Subsystem7/RConn1
  Half-Bridge MMC Bm (Aggregate model of 36 PM)1/LConn2 -- Subsystem9/LConn2
  Half-Bridge MMC Am (Aggregate model of 36 PM)1/LConn2 -- Subsystem7/LConn2
  Subsystem8/RConn2 -- Series RLC Branch20/LConn1
  Half-Bridge MMC Cm (Aggregate model of 36 PM)1/LConn2 -- Subsystem11/LConn2
  Series RLC Branch17/RConn1 -- Subsystem9/RConn1
  Half-Bridge MMC Am (Aggregate model of 36 PM)1/LConn1 -- Subsystem7/LConn1
  Half-Bridge MMC Cp (Aggregate model of 36 PM)1/LConn2 -- Subsystem10/LConn2
  Half-Bridge MMC Bp (Aggregate model of 36 PM) 1/LConn1 -- Subsystem8/LConn1
  Series RLC Branch24/RConn1 -- Subsystem11/RConn1
  Subsystem10/RConn2 -- Series RLC Branch16/LConn1
  Half-Bridge MMC Cp (Aggregate model of 36 PM)1/LConn1 -- Subsystem10/LConn1
  Subsystem6/RConn2 -- Series RLC Branch23/LConn1
  prim1/RConn1 -- DFIG Wind Turbine/LConn1
  DFIG Wind Turbine/LConn2 -- prim1/RConn2
  DFIG Wind Turbine/LConn3 -- prim1/RConn3
  Brk3/LConn1 -- prim2/LConn1
  prim2/LConn2 -- Brk3/LConn2
  prim2/LConn3 -- Brk3/LConn3
  DC & converter 2/RConn2 -- DC & converter 1/RConn2
  Tr2/RConn1 -- prim2/RConn1
  Tr2/RConn2 -- prim2/RConn2
  Tr2/LConn3 -- prim1/LConn3
  Tr2/LConn2 -- prim1/LConn2
  Tr2/LConn1 -- prim1/LConn1
  Tr2/RConn3 -- prim2/RConn3
  DC & converter 2/LConn2 -- Subsystem1/RConn2 -- Subsystem3/RConn2 -- Subsystem5/RConn2
  Series RLC Branch4/RConn1 -- Series RLC Branch3/LConn1 -- Current Measurement2/RConn1
  Series RLC Branch11/RConn1 -- Current Measurement1/RConn1 -- Series RLC Branch10/LConn1
  Three-Phase Fault/LConn1 -- sec/LConn1 -- Current Measurement/LConn1
  Subsystem/RConn1 -- Subsystem2/RConn1 -- Current Measurement3/RConn1 -- Subsystem4/RConn1
  DC & converter 2/RConn1 -- DC & converter 1/RConn1
  Current Measurement3/LConn1 -- DC & converter 2/LConn1
